simulink library "xps_library"  (R2018a)
settings: Solver=ode45  StartTime=0.0  StopTime=10.0  RelTol=1e-3
undefined symbols (not defined in the file or in its folder): ip_name, lib_path
libraries: xbsIndex_r4 x2454, casper_library_flow_control x68, simulink x52, $bdroot x22, casper_library_misc x9
(part 15 of 27)

== system xps_library/Memory/hmc/sim_mem1 ==
  rd_en : Inport
  wr_en : Inport  Port=2
  wr_addr : Inport  Port=3
  data : Inport  Port=4
  rd_addr : Inport  Port=5
  rd_tag : Inport  Port=6
  Data Type Conversion : DataTypeConversion  OutDataTypeStr=single
  Data Type Conversion2 : DataTypeConversion  OutDataTypeStr=boolean
  Data Type Conversion3 : DataTypeConversion  OutDataTypeStr=single
  Data Type Conversion4 : DataTypeConversion  OutDataTypeStr=boolean
  Data Type Conversion5 : DataTypeConversion  OutDataTypeStr=single
  bus_create : Subsystem  AncestorBlock=casper_library_flow_control/bus_create  mask(bus_create){inputNum=8}
      mask prompts: inputNum "Number of inputs:"
      mask init:
      | bus_create_init(gcb,...
      |     'inputNum', inputNum);
  bus_expand : Subsystem  AncestorBlock=casper_library_flow_control/bus_expand  mask(bus_expand){mode=divisions of equal size, outputNum=8, outputWidth=32, outputBinaryPt=0, outputArithmeticType=0, show_format=off, outputToWorkspace=off, variablePrefix=out, outputToModelAsWell=on}
      mask prompts: outputNum "Number of outputs:"; outputWidth "Output width:"; outputBinaryPt "Output binary point position:"; outputArithmeticType "Output arithmetic type (ufix=0, fix=1, bool=2):"; show_format "Print format string?"; outputToWorkspace "Output to workspace?"; variablePrefix "Variable name prefix:"; outputToModelAsWell "Output to model as well?"
      mask help:
      | Expands a 'bus' made using a bus_create or Xilinx
      | concat block.
      | The input will be divided into the specified number
      | of outputs with the specified arithmetic types.
      | Divisions are made from most significant bit.
      mask init: same as xps_library/IO/forty_gbe/rx_dv_or_exp
      settings: AttributesFormatString=8 outputs
      mask TypeOptions mode: divisions of equal size | divisions of arbitrary size
      mask Callback mode: bus_expand_callback();
      mask Callback outputWidth: bus_expand_callback();
      mask Callback outputToWorkspace: bus_expand_callback();
  data_to_xilinx{1..8} (8 alike) : xbsIndex_r4/Gateway In  gui_display_data_type=Fixed-point  arith_type=Unsigned  n_bits=32  bin_pt=0  preci_type=Single  exp_width=8  frac_width=24  rows=1  columns=1  quantization="Round  (unbiased: +/- Inf)"  overflow=Saturate  period=1  UseAsADC=off  ADCChannel='1'  interface=None  automatic_assignment=on  address_offset=hex2dec('00')  intf_name=''  intf_description=''  default_value=0  timing_constraint=None  locs_specified=off  LOCs={}  io_standard={}  inherit_from_input=off  hdl_port=on  dbl_ovrd=off  block_type=gatewayin
  gateway_data_out : xbsIndex_r4/Gateway Out  inherit_from_input=off  hdl_port=off  rows=1  columns=1  UseAsDAC=off  DACChannel='1'  interface=None  automatic_assignment=on  address_offset=hex2dec('00')  intf_name=''  intf_description=''  timing_constraint=None  locs_specified=off  LOCs={}  io_standard={}  block_type=gatewayout
  sfunc : M-S-Function  FunctionName=hmc_sim_sfunc  Parameters=depth_bits, latency, randread  mask{depth_bits=addr_width, latency=csp_latency, randread=on}
      mask prompts: depth_bits "Depth (2^?):"; latency "Latency (>=1):"; randread "Randomise read results"
      mask init:
      | % if randread
      | %     sprintf('sfunc randread 1')
      | % else
      | %     sprintf('sfunc randread 0')
      | % end
      mask Callback latency:
      | latency = str2double(get_param(gcb, 'latency'));
      | if latency < 1
      |     errordlg('Cannot have latency less than one.');
      |     set_param(gcb, 'latency', '1');
      | end
  sim_data_0_31 : xbsIndex_r4/Gateway Out  inherit_from_input=off  hdl_port=off  rows=1  columns=1  UseAsDAC=off  DACChannel='1'  interface=None  automatic_assignment=on  address_offset=hex2dec('00')  intf_name=''  intf_description=''  timing_constraint=None  locs_specified=off  LOCs={}  io_standard={}  block_type=gatewayout
  sim_data_128_159 : xbsIndex_r4/Gateway Out  inherit_from_input=off  hdl_port=off  rows=1  columns=1  UseAsDAC=off  DACChannel='1'  interface=None  automatic_assignment=on  address_offset=hex2dec('00')  intf_name=''  intf_description=''  timing_constraint=None  locs_specified=off  LOCs={}  io_standard={}  block_type=gatewayout
  sim_data_160_191 : xbsIndex_r4/Gateway Out  inherit_from_input=off  hdl_port=off  rows=1  columns=1  UseAsDAC=off  DACChannel='1'  interface=None  automatic_assignment=on  address_offset=hex2dec('00')  intf_name=''  intf_description=''  timing_constraint=None  locs_specified=off  LOCs={}  io_standard={}  block_type=gatewayout
  sim_data_192_223 : xbsIndex_r4/Gateway Out  inherit_from_input=off  hdl_port=off  rows=1  columns=1  UseAsDAC=off  DACChannel='1'  interface=None  automatic_assignment=on  address_offset=hex2dec('00')  intf_name=''  intf_description=''  timing_constraint=None  locs_specified=off  LOCs={}  io_standard={}  block_type=gatewayout
  sim_data_224_255 : xbsIndex_r4/Gateway Out  inherit_from_input=off  hdl_port=off  rows=1  columns=1  UseAsDAC=off  DACChannel='1'  interface=None  automatic_assignment=on  address_offset=hex2dec('00')  intf_name=''  intf_description=''  timing_constraint=None  locs_specified=off  LOCs={}  io_standard={}  block_type=gatewayout
  sim_data_32_63 : xbsIndex_r4/Gateway Out  inherit_from_input=off  hdl_port=off  rows=1  columns=1  UseAsDAC=off  DACChannel='1'  interface=None  automatic_assignment=on  address_offset=hex2dec('00')  intf_name=''  intf_description=''  timing_constraint=None  locs_specified=off  LOCs={}  io_standard={}  block_type=gatewayout
  sim_data_64_95 : xbsIndex_r4/Gateway Out  inherit_from_input=off  hdl_port=off  rows=1  columns=1  UseAsDAC=off  DACChannel='1'  interface=None  automatic_assignment=on  address_offset=hex2dec('00')  intf_name=''  intf_description=''  timing_constraint=None  locs_specified=off  LOCs={}  io_standard={}  block_type=gatewayout
  sim_data_96_127 : xbsIndex_r4/Gateway Out  inherit_from_input=off  hdl_port=off  rows=1  columns=1  UseAsDAC=off  DACChannel='1'  interface=None  automatic_assignment=on  address_offset=hex2dec('00')  intf_name=''  intf_description=''  timing_constraint=None  locs_specified=off  LOCs={}  io_standard={}  block_type=gatewayout
  sim_rd_addr : xbsIndex_r4/Gateway Out  inherit_from_input=off  hdl_port=off  rows=1  columns=1  UseAsDAC=off  DACChannel='1'  interface=None  automatic_assignment=on  address_offset=hex2dec('00')  intf_name=''  intf_description=''  timing_constraint=None  locs_specified=off  LOCs={}  io_standard={}  block_type=gatewayout
  sim_rd_en : xbsIndex_r4/Gateway Out  inherit_from_input=off  hdl_port=off  rows=1  columns=1  UseAsDAC=off  DACChannel='1'  interface=None  automatic_assignment=on  address_offset=hex2dec('00')  intf_name=''  intf_description=''  timing_constraint=None  locs_specified=off  LOCs={}  io_standard={}  block_type=gatewayout
  sim_rd_tag : xbsIndex_r4/Gateway Out  inherit_from_input=off  hdl_port=off  rows=1  columns=1  UseAsDAC=off  DACChannel='1'  interface=None  automatic_assignment=on  address_offset=hex2dec('00')  intf_name=''  intf_description=''  timing_constraint=None  locs_specified=off  LOCs={}  io_standard={}  block_type=gatewayout
  sim_rw_addr : xbsIndex_r4/Gateway Out  inherit_from_input=off  hdl_port=off  rows=1  columns=1  UseAsDAC=off  DACChannel='1'  interface=None  automatic_assignment=on  address_offset=hex2dec('00')  intf_name=''  intf_description=''  timing_constraint=None  locs_specified=off  LOCs={}  io_standard={}  block_type=gatewayout
  sim_wr_en : xbsIndex_r4/Gateway Out  inherit_from_input=off  hdl_port=off  rows=1  columns=1  UseAsDAC=off  DACChannel='1'  interface=None  automatic_assignment=on  address_offset=hex2dec('00')  intf_name=''  intf_description=''  timing_constraint=None  locs_specified=off  LOCs={}  io_standard={}  block_type=gatewayout
  data_out : Outport
  dv_out : Outport  Port=2
  tag_out : Outport  Port=3
  wires:
  bus_expand/8(lsb_out1) -> sim_data_224_255/1
  bus_expand/7(out2) -> sim_data_192_223/1
  bus_expand/6(out3) -> sim_data_160_191/1
  bus_expand/5(out4) -> sim_data_128_159/1
  bus_expand/4(out5) -> sim_data_96_127/1
  bus_expand/3(out6) -> sim_data_64_95/1
  bus_expand/2(out7) -> sim_data_32_63/1
  bus_expand/1(msb_out8) -> sim_data_0_31/1
  rd_tag/1 -> sim_rd_tag/1
  sim_rd_tag/1 -> Data Type Conversion3/1
  rd_addr/1 -> sim_rd_addr/1
  sim_rd_addr/1 -> Data Type Conversion5/1
  rd_en/1 -> sim_rd_en/1
  sim_rd_en/1 -> Data Type Conversion4/1
  Data Type Conversion4/1 -> sfunc/1  "rd_en"
  wr_addr/1 -> sim_rw_addr/1
  wr_en/1 -> sim_wr_en/1
  sim_rw_addr/1 -> Data Type Conversion/1
  sim_wr_en/1 -> Data Type Conversion2/1
  Data Type Conversion/1 -> sfunc/3  "wr_addr"
  Data Type Conversion2/1 -> sfunc/2  "wr_en"
  Data Type Conversion5/1 -> sfunc/12  "rd_addr"
  Data Type Conversion3/1 -> sfunc/13  "rd_tag"
  data/1 -> bus_expand/1(bus_in)
  sim_data_224_255/1 -> sfunc/11
  sim_data_192_223/1 -> sfunc/10
  sim_data_160_191/1 -> sfunc/9
  sim_data_128_159/1 -> sfunc/8
  sim_data_96_127/1 -> sfunc/7
  sim_data_64_95/1 -> sfunc/6
  sim_data_32_63/1 -> sfunc/5
  sim_data_0_31/1 -> sfunc/4
  bus_create/1(bus_out) -> gateway_data_out/1
  gateway_data_out/1 -> data_out/1
  data_to_xilinx1/1 -> bus_create/1(in1)
  data_to_xilinx2/1 -> bus_create/2(in2)
  data_to_xilinx3/1 -> bus_create/3(in3)
  data_to_xilinx5/1 -> bus_create/5(in5)
  data_to_xilinx6/1 -> bus_create/6(in6)
  data_to_xilinx7/1 -> bus_create/7(in7)
  data_to_xilinx8/1 -> bus_create/8(in8)
  data_to_xilinx4/1 -> bus_create/4(in4)
  sfunc/1 -> data_to_xilinx1/1  "output"
  sfunc/2 -> data_to_xilinx2/1
  sfunc/3 -> data_to_xilinx3/1
  sfunc/4 -> data_to_xilinx4/1
  sfunc/5 -> data_to_xilinx5/1
  sfunc/6 -> data_to_xilinx6/1
  sfunc/7 -> data_to_xilinx7/1
  sfunc/8 -> data_to_xilinx8/1
  sfunc/9 -> dv_out/1
  sfunc/10 -> tag_out/1

== system xps_library/Memory/hmc/sim_mem2 ==
  rd_en : Inport
  wr_en : Inport  Port=2
  wr_addr : Inport  Port=3
  data : Inport  Port=4
  rd_addr : Inport  Port=5
  rd_tag : Inport  Port=6
  Data Type Conversion : DataTypeConversion  OutDataTypeStr=single
  Data Type Conversion2 : DataTypeConversion  OutDataTypeStr=boolean
  Data Type Conversion3 : DataTypeConversion  OutDataTypeStr=single
  Data Type Conversion4 : DataTypeConversion  OutDataTypeStr=boolean
  Data Type Conversion5 : DataTypeConversion  OutDataTypeStr=single
  bus_create : Subsystem  AncestorBlock=casper_library_flow_control/bus_create  mask(bus_create){inputNum=8}
      mask prompts: inputNum "Number of inputs:"
      mask init:
      | bus_create_init(gcb,...
      |     'inputNum', inputNum);
  bus_expand : Subsystem  AncestorBlock=casper_library_flow_control/bus_expand  mask(bus_expand){mode=divisions of equal size, outputNum=8, outputWidth=32, outputBinaryPt=0, outputArithmeticType=0, show_format=off, outputToWorkspace=off, variablePrefix=out, outputToModelAsWell=on}
      mask prompts: outputNum "Number of outputs:"; outputWidth "Output width:"; outputBinaryPt "Output binary point position:"; outputArithmeticType "Output arithmetic type (ufix=0, fix=1, bool=2):"; show_format "Print format string?"; outputToWorkspace "Output to workspace?"; variablePrefix "Variable name prefix:"; outputToModelAsWell "Output to model as well?"
      mask help:
      | Expands a 'bus' made using a bus_create or Xilinx
      | concat block.
      | The input will be divided into the specified number
      | of outputs with the specified arithmetic types.
      | Divisions are made from most significant bit.
      mask init: same as xps_library/IO/forty_gbe/rx_dv_or_exp
      settings: AttributesFormatString=8 outputs
      mask TypeOptions mode: divisions of equal size | divisions of arbitrary size
      mask Callback mode: bus_expand_callback();
      mask Callback outputWidth: bus_expand_callback();
      mask Callback outputToWorkspace: bus_expand_callback();
  data_to_xilinx{1..8} (8 alike) : xbsIndex_r4/Gateway In  gui_display_data_type=Fixed-point  arith_type=Unsigned  n_bits=32  bin_pt=0  preci_type=Single  exp_width=8  frac_width=24  rows=1  columns=1  quantization="Round  (unbiased: +/- Inf)"  overflow=Saturate  period=1  UseAsADC=off  ADCChannel='1'  interface=None  automatic_assignment=on  address_offset=hex2dec('00')  intf_name=''  intf_description=''  default_value=0  timing_constraint=None  locs_specified=off  LOCs={}  io_standard={}  inherit_from_input=off  hdl_port=on  dbl_ovrd=off  block_type=gatewayin
  gateway_data_out : xbsIndex_r4/Gateway Out  inherit_from_input=off  hdl_port=off  rows=1  columns=1  UseAsDAC=off  DACChannel='1'  interface=None  automatic_assignment=on  address_offset=hex2dec('00')  intf_name=''  intf_description=''  timing_constraint=None  locs_specified=off  LOCs={}  io_standard={}  block_type=gatewayout
  sfunc : M-S-Function  FunctionName=hmc_sim_sfunc  Parameters=depth_bits, latency, randread  mask{depth_bits=addr_width, latency=csp_latency, randread=on}
      mask prompts: depth_bits "Depth (2^?):"; latency "Latency (>=1):"; randread "Randomise read results"
      mask Callback latency:
      | latency = str2double(get_param(gcb, 'latency'));
      | if latency < 1
      |     errordlg('Cannot have latency less than one.');
      |     set_param(gcb, 'latency', '1');
      | end
  sim_data_0_31 : xbsIndex_r4/Gateway Out  inherit_from_input=off  hdl_port=off  rows=1  columns=1  UseAsDAC=off  DACChannel='1'  interface=None  automatic_assignment=on  address_offset=hex2dec('00')  intf_name=''  intf_description=''  timing_constraint=None  locs_specified=off  LOCs={}  io_standard={}  block_type=gatewayout
  sim_data_128_159 : xbsIndex_r4/Gateway Out  inherit_from_input=off  hdl_port=off  rows=1  columns=1  UseAsDAC=off  DACChannel='1'  interface=None  automatic_assignment=on  address_offset=hex2dec('00')  intf_name=''  intf_description=''  timing_constraint=None  locs_specified=off  LOCs={}  io_standard={}  block_type=gatewayout
  sim_data_160_191 : xbsIndex_r4/Gateway Out  inherit_from_input=off  hdl_port=off  rows=1  columns=1  UseAsDAC=off  DACChannel='1'  interface=None  automatic_assignment=on  address_offset=hex2dec('00')  intf_name=''  intf_description=''  timing_constraint=None  locs_specified=off  LOCs={}  io_standard={}  block_type=gatewayout
  sim_data_192_223 : xbsIndex_r4/Gateway Out  inherit_from_input=off  hdl_port=off  rows=1  columns=1  UseAsDAC=off  DACChannel='1'  interface=None  automatic_assignment=on  address_offset=hex2dec('00')  intf_name=''  intf_description=''  timing_constraint=None  locs_specified=off  LOCs={}  io_standard={}  block_type=gatewayout
  sim_data_224_255 : xbsIndex_r4/Gateway Out  inherit_from_input=off  hdl_port=off  rows=1  columns=1  UseAsDAC=off  DACChannel='1'  interface=None  automatic_assignment=on  address_offset=hex2dec('00')  intf_name=''  intf_description=''  timing_constraint=None  locs_specified=off  LOCs={}  io_standard={}  block_type=gatewayout
  sim_data_32_63 : xbsIndex_r4/Gateway Out  inherit_from_input=off  hdl_port=off  rows=1  columns=1  UseAsDAC=off  DACChannel='1'  interface=None  automatic_assignment=on  address_offset=hex2dec('00')  intf_name=''  intf_description=''  timing_constraint=None  locs_specified=off  LOCs={}  io_standard={}  block_type=gatewayout
  sim_data_64_95 : xbsIndex_r4/Gateway Out  inherit_from_input=off  hdl_port=off  rows=1  columns=1  UseAsDAC=off  DACChannel='1'  interface=None  automatic_assignment=on  address_offset=hex2dec('00')  intf_name=''  intf_description=''  timing_constraint=None  locs_specified=off  LOCs={}  io_standard={}  block_type=gatewayout
  sim_data_96_127 : xbsIndex_r4/Gateway Out  inherit_from_input=off  hdl_port=off  rows=1  columns=1  UseAsDAC=off  DACChannel='1'  interface=None  automatic_assignment=on  address_offset=hex2dec('00')  intf_name=''  intf_description=''  timing_constraint=None  locs_specified=off  LOCs={}  io_standard={}  block_type=gatewayout
  sim_rd_addr : xbsIndex_r4/Gateway Out  inherit_from_input=off  hdl_port=off  rows=1  columns=1  UseAsDAC=off  DACChannel='1'  interface=None  automatic_assignment=on  address_offset=hex2dec('00')  intf_name=''  intf_description=''  timing_constraint=None  locs_specified=off  LOCs={}  io_standard={}  block_type=gatewayout
  sim_rd_en : xbsIndex_r4/Gateway Out  inherit_from_input=off  hdl_port=off  rows=1  columns=1  UseAsDAC=off  DACChannel='1'  interface=None  automatic_assignment=on  address_offset=hex2dec('00')  intf_name=''  intf_description=''  timing_constraint=None  locs_specified=off  LOCs={}  io_standard={}  block_type=gatewayout
  sim_rd_tag : xbsIndex_r4/Gateway Out  inherit_from_input=off  hdl_port=off  rows=1  columns=1  UseAsDAC=off  DACChannel='1'  interface=None  automatic_assignment=on  address_offset=hex2dec('00')  intf_name=''  intf_description=''  timing_constraint=None  locs_specified=off  LOCs={}  io_standard={}  block_type=gatewayout
  sim_rw_addr : xbsIndex_r4/Gateway Out  inherit_from_input=off  hdl_port=off  rows=1  columns=1  UseAsDAC=off  DACChannel='1'  interface=None  automatic_assignment=on  address_offset=hex2dec('00')  intf_name=''  intf_description=''  timing_constraint=None  locs_specified=off  LOCs={}  io_standard={}  block_type=gatewayout
  sim_wr_en : xbsIndex_r4/Gateway Out  inherit_from_input=off  hdl_port=off  rows=1  columns=1  UseAsDAC=off  DACChannel='1'  interface=None  automatic_assignment=on  address_offset=hex2dec('00')  intf_name=''  intf_description=''  timing_constraint=None  locs_specified=off  LOCs={}  io_standard={}  block_type=gatewayout
  data_out : Outport
  dv_out : Outport  Port=2
  tag_out : Outport  Port=3
  wires:
  bus_expand/8(lsb_out1) -> sim_data_224_255/1
  bus_expand/7(out2) -> sim_data_192_223/1
  bus_expand/6(out3) -> sim_data_160_191/1
  bus_expand/5(out4) -> sim_data_128_159/1
  bus_expand/4(out5) -> sim_data_96_127/1
  bus_expand/3(out6) -> sim_data_64_95/1
  bus_expand/2(out7) -> sim_data_32_63/1
  bus_expand/1(msb_out8) -> sim_data_0_31/1
  rd_tag/1 -> sim_rd_tag/1
  sim_rd_tag/1 -> Data Type Conversion3/1
  rd_addr/1 -> sim_rd_addr/1
  sim_rd_addr/1 -> Data Type Conversion5/1
  rd_en/1 -> sim_rd_en/1
  sim_rd_en/1 -> Data Type Conversion4/1
  Data Type Conversion4/1 -> sfunc/1  "rd_en"
  wr_addr/1 -> sim_rw_addr/1
  wr_en/1 -> sim_wr_en/1
  sim_rw_addr/1 -> Data Type Conversion/1
  sim_wr_en/1 -> Data Type Conversion2/1
  Data Type Conversion/1 -> sfunc/3  "wr_addr"
  Data Type Conversion2/1 -> sfunc/2  "wr_en"
  Data Type Conversion5/1 -> sfunc/12  "rd_addr"
  Data Type Conversion3/1 -> sfunc/13  "rd_tag"
  data/1 -> bus_expand/1(bus_in)
  sim_data_224_255/1 -> sfunc/11
  sim_data_192_223/1 -> sfunc/10
  sim_data_160_191/1 -> sfunc/9
  sim_data_128_159/1 -> sfunc/8
  sim_data_96_127/1 -> sfunc/7
  sim_data_64_95/1 -> sfunc/6
  sim_data_32_63/1 -> sfunc/5
  sim_data_0_31/1 -> sfunc/4
  gateway_data_out/1 -> data_out/1
  bus_create/1(bus_out) -> gateway_data_out/1
  data_to_xilinx1/1 -> bus_create/1(in1)
  data_to_xilinx2/1 -> bus_create/2(in2)
  data_to_xilinx3/1 -> bus_create/3(in3)
  data_to_xilinx5/1 -> bus_create/5(in5)
  data_to_xilinx6/1 -> bus_create/6(in6)
  data_to_xilinx7/1 -> bus_create/7(in7)
  data_to_xilinx8/1 -> bus_create/8(in8)
  data_to_xilinx4/1 -> bus_create/4(in4)
  sfunc/1 -> data_to_xilinx1/1  "output"
  sfunc/2 -> data_to_xilinx2/1
  sfunc/3 -> data_to_xilinx3/1
  sfunc/4 -> data_to_xilinx4/1
  sfunc/5 -> data_to_xilinx5/1
  sfunc/6 -> data_to_xilinx6/1
  sfunc/7 -> data_to_xilinx7/1
  sfunc/8 -> data_to_xilinx8/1
  sfunc/9 -> dv_out/1
  sfunc/10 -> tag_out/1

== system xps_library/Memory/qdr/qdr_sim_model ==
  rd_en : Inport
  wr_en : Inport  Port=2
  be : Inport  Port=3
  addr : Inport  Port=4
  data_in : Inport  Port=5
  AddSub : xbsIndex_r4/AddSub  mode=Addition  use_carryin=off  use_carryout=off  en=off  latency=0  precision=Full  arith_type=Unsigned  n_bits=16  bin_pt=14  quantization=Truncate  overflow=Wrap  use_behavioral_HDL=off  hw_selection=Fabric  pipelined=off  use_rpm=on  dbl_ovrd=off  block_type=addsub
      settings: block_version=10.1.3
  Concat : xbsIndex_r4/Concat  num_inputs=2  dbl_ovrd=off  block_type=concat
      settings: block_version=10.1.3
  Constant1 : xbsIndex_r4/Constant  const=0  gui_display_data_type=Fixed-point  arith_type=Unsigned  n_bits=1  bin_pt=0  preci_type=Single  exp_width=8  frac_width=24  explicit_period=on  period=1  equ=P=C  opselect=C  inp2=PCIN>>17  opr=+  inp1=P  carry=CIN  dbl_ovrd=off  block_type=constant
  Constant2 : xbsIndex_r4/Constant  const=1  gui_display_data_type=Fixed-point  arith_type=Unsigned  n_bits=33  bin_pt=0  preci_type=Single  exp_width=8  frac_width=24  explicit_period=on  period=1  equ=P=C  opselect=C  inp2=PCIN>>17  opr=+  inp1=P  carry=CIN  dbl_ovrd=off  block_type=constant
  Delay : xbsIndex_r4/Delay  rst=off  infoeditControl=Selection of Reset will increase slice count due to use of real FFs and instead of SRLs  en=off  latency=9  reg_retiming=off  dbl_ovrd=off  block_type=delay
  Delay{1..3,5} (4 alike) : xbsIndex_r4/Delay  rst=off  infoeditControl=Selection of Reset will increase slice count due to use of real FFs and instead of SRLs  en=off  latency=1  reg_retiming=off  dbl_ovrd=off  block_type=delay
  Delay4 : xbsIndex_r4/Delay  rst=off  infoeditControl=Selection of Reset will increase slice count due to use of real FFs and instead of SRLs  en=off  latency=10  reg_retiming=off  dbl_ovrd=off  block_type=delay
  Dual Port RAM : xbsIndex_r4/Dual Port RAM  depth=2^qdr_awidth  initVector=[1:2^qdr_awidth]  distributed_mem=Block RAM  init_a=0  init_b=0  rst_a=off  rst_b=off  en_a=off  en_b=off  latency=1  write_mode_A=Read After Write  write_mode_B=Read After Write  optimize=Area  dbl_ovrd=off  block_type=dpram
      settings: block_version=10.1.3
  Inverter1 : xbsIndex_r4/Inverter  en=off  latency=0  dbl_ovrd=off  block_type=inv
  Inverter2 : xbsIndex_r4/Inverter  en=off  latency=0  dbl_ovrd=off  block_type=inv
  Inverter3 : xbsIndex_r4/Inverter  en=off  latency=0  dbl_ovrd=off  block_type=inv
  Logical : xbsIndex_r4/Logical  logical_function=AND  inputs=2  en=off  latency=0  precision=Full  arith_type=Unsigned  n_bits=16  bin_pt=0  align_bp=on  dbl_ovrd=off  block_type=logical
  Logical1 : xbsIndex_r4/Logical  logical_function=AND  inputs=2  en=off  latency=0  precision=Full  arith_type=Unsigned  n_bits=16  bin_pt=0  align_bp=on  dbl_ovrd=off  block_type=logical
  Logical2 : xbsIndex_r4/Logical  logical_function=AND  inputs=2  en=off  latency=0  precision=Full  arith_type=Unsigned  n_bits=16  bin_pt=0  align_bp=on  dbl_ovrd=off  block_type=logical
  Logical3 : xbsIndex_r4/Logical  logical_function=OR  inputs=2  en=off  latency=0  precision=Full  arith_type=Unsigned  n_bits=16  bin_pt=0  align_bp=on  dbl_ovrd=off  block_type=logical
  Mux : xbsIndex_r4/Mux  inputs=2  en=off  latency=0  precision=Full  arith_type=Unsigned  n_bits=16  bin_pt=14  quantization=Truncate  overflow=Wrap  dbl_ovrd=off  block_type=mux
  Terminator : Terminator
  convert_address : xbsIndex_r4/Convert  gui_display_data_type=Fixed-point  arith_type=Unsigned  n_bits=qdr_awidth  bin_pt=0  float_type=Single  exp_bits=8  fraction_bits=24  quantization=Truncate  overflow=Wrap  en=off  latency=0  pipeline=off  dbl_ovrd=off  block_type=convert
      settings: xl_area=[0, 0, 0, 0, 0, 0, 0]
  convert_address1 : xbsIndex_r4/Convert  gui_display_data_type=Fixed-point  arith_type=Unsigned  n_bits=qdr_awidth  bin_pt=0  float_type=Single  exp_bits=8  fraction_bits=24  quantization=Truncate  overflow=Wrap  en=off  latency=0  pipeline=off  dbl_ovrd=off  block_type=convert
      settings: xl_area=[0, 0, 0, 0, 0, 0, 0]
  prev_rd : xbsIndex_r4/Register  init=0  rst=off  en=off  dbl_ovrd=off  block_type=register
  prev_w : xbsIndex_r4/Register  init=0  rst=off  en=off  dbl_ovrd=off  block_type=register
  sim_data_out : xbsIndex_r4/Gateway Out  inherit_from_input=off  hdl_port=off  rows=1  columns=1  UseAsDAC=off  DACChannel='1'  interface=None  automatic_assignment=on  address_offset=hex2dec('00')  intf_name=''  intf_description=''  timing_constraint=None  locs_specified=off  LOCs={'B21','B22','A22','B23','B19','C19','A20','A21','A23','B24','A24','A25','E18','D18','C18','B18'}  io_standard={}  block_type=gatewayout
      settings: sginterface={'Nallatech'=>{'xdspkit'=>{'non_memory_mapped_port'=>'sim_data_out'}},'Xilinx'=>{'jtaghwcosim'=>{'non_memory_mapped_port'=>'sim_data_out'},'xdspkit'=>{'non_memory_mapped_port'=>'sim_data_out'}}}  xl_area=[0, 0, 0, 0, 0, 0, 0]
  sim_data_vld : xbsIndex_r4/Gateway Out  inherit_from_input=off  hdl_port=off  rows=1  columns=1  UseAsDAC=off  DACChannel='1'  interface=None  automatic_assignment=on  address_offset=hex2dec('00')  intf_name=''  intf_description=''  timing_constraint=None  locs_specified=off  LOCs={'B21','B22','A22','B23','B19','C19','A20','A21','A23','B24','A24','A25','E18','D18','C18','B18'}  io_standard={}  block_type=gatewayout
      settings: sginterface={'Nallatech'=>{'xdspkit'=>{'non_memory_mapped_port'=>'sim_data_out'}},'Xilinx'=>{'jtaghwcosim'=>{'non_memory_mapped_port'=>'sim_data_out'},'xdspkit'=>{'non_memory_mapped_port'=>'sim_data_out'}}}  xl_area=[0, 0, 0, 0, 0, 0, 0]
  data_out : Outport
  data_valid : Outport  Port=2
  wires:
  Dual Port RAM/2 -> Mux/2
  Dual Port RAM/1 -> Mux/3
  Delay3/1 -> Mux/1
  [R] -> Delay3/1
  Mux/1 -> Delay/1
  Inverter1/1 -> Logical1/2
  Inverter3/1 -> Logical2/2
  Logical2/1 -> prev_w/1, [W]
  prev_w/1 -> Inverter3/1
  Logical1/1 -> Logical2/1
  [W] -> Delay1/1
  [W] -> Dual Port RAM/3
  [A] -> convert_address/1
  [Az] -> convert_address1/1
  [D] -> Dual Port RAM/2
  data_in/1 -> [D]
  [R] -> Inverter1/1
  wr_en/1 -> Logical1/1
  Logical/1 -> [R], prev_rd/1
  Inverter2/1 -> Logical/2
  prev_rd/1 -> Inverter2/1
  rd_en/1 -> Delay4/1, Logical/1
  AddSub/1 -> [Az]
  Constant2/1 -> AddSub/2
  Delay2/1 -> AddSub/1
  Concat/1 -> [A], Delay2/1
  Constant1/1 -> Concat/2
  addr/1 -> Concat/1
  Delay1/1 -> Dual Port RAM/6
  [D] -> Dual Port RAM/5
  convert_address/1 -> Dual Port RAM/1
  convert_address1/1 -> Dual Port RAM/4
  sim_data_out/1 -> data_out/1
  Delay/1 -> sim_data_out/1
  be/1 -> Terminator/1
  sim_data_vld/1 -> data_valid/1
  Delay4/1 -> Delay5/1, Logical3/1
  Delay5/1 -> Logical3/2
  Logical3/1 -> sim_data_vld/1

== system xps_library/Memory/shared_bram/calc_add ==
  note: If reading/writing words
      | smaller than 32 bits,
      | change address so
      | that addressing is
      | big endian instead of
      | little, otherwise
      | pass through
  note: Use behavioural HDL
      | so that gets optimised
      | to minimum logic
  in : Inport
  add_sub : xbsIndex_r4/AddSub  mode=Subtraction  use_carryin=off  use_carryout=off  en=off  latency=0  precision=User Defined  arith_type=Unsigned  n_bits=max(1, log2(32/data_width))  bin_pt=0  quantization=Truncate  overflow=Wrap  use_behavioral_HDL=on  hw_selection=Fabric  pipelined=off  dbl_ovrd=off  block_type=addsub
  concat : xbsIndex_r4/Concat  num_inputs=2  dbl_ovrd=off  block_type=concat
  const : xbsIndex_r4/Constant  const=max(0, 32/data_width-1)  gui_display_data_type=Fixed-point  arith_type=Unsigned  n_bits=max(1, log2(32/data_width))  bin_pt=0  preci_type=Single  exp_width=8  frac_width=24  explicit_period=on  period=sample_rate  equ=P=C  opselect=C  inp2=PCIN>>17  opr=+  inp1=P  carry=CIN  dbl_ovrd=off  block_type=constant
      settings: block_version=11.4
  convert_addr : xbsIndex_r4/Convert  gui_display_data_type=Fixed-point  arith_type=Unsigned  n_bits=addr_width  bin_pt=0  float_type=Single  exp_bits=8  fraction_bits=24  quantization=Truncate  overflow=Wrap  en=off  latency=0  pipeline=off  dbl_ovrd=off  block_type=convert
      settings: xl_area=[0, 0, 0, 0, 0, 0, 0]
  lsw : xbsIndex_r4/Slice  nbits=max(1, log2(32/data_width))  boolean_output=off  mode=Lower Bit Location + Width  bit1=0  base1=MSB of Input  bit0=0  base0=LSB of Input  dbl_ovrd=off  block_type=slice
  manipulate : xbsIndex_r4/Constant  const=min(1, floor(32/data_width) - 1)  gui_display_data_type=Fixed-point  arith_type=Unsigned  n_bits=1  bin_pt=0  preci_type=Single  exp_width=8  frac_width=24  explicit_period=on  period=sample_rate  equ=P=C  opselect=C  inp2=PCIN>>17  opr=+  inp1=P  carry=CIN  dbl_ovrd=off  block_type=constant
      settings: block_version=11.4
  msw : xbsIndex_r4/Slice  nbits=addr_width - max(1, log2(32/data_width))  boolean_output=off  mode=Upper Bit Location + Width  bit1=0  base1=MSB of Input  bit0=0  base0=LSB of Input  dbl_ovrd=off  block_type=slice
  mux : xbsIndex_r4/Mux  inputs=2  en=off  latency=0  precision=Full  arith_type=Unsigned  n_bits=16  bin_pt=14  quantization=Truncate  overflow=Wrap  dbl_ovrd=off  block_type=mux
      settings: block_version=11.4
  out : Outport
  wires:
  in/1 -> convert_addr/1
  add_sub/1 -> concat/2
  msw/1 -> concat/1
  concat/1 -> mux/3
  manipulate/1 -> mux/1
  mux/1 -> out/1
  lsw/1 -> add_sub/2
  const/1 -> add_sub/1
  convert_addr/1 -> lsw/1, msw/1, mux/2

== system xps_library/Memory/shared_bram/munge_in ==
  din : Inport
  reinterpret_out : xbsIndex_r4/Reinterpret  force_arith_type=on  arith_type=Unsigned  force_bin_pt=on  bin_pt=0  block_type=reinterpret
  dout : Outport
  wires:
  reinterpret_out/1 -> dout/1
  din/1 -> reinterpret_out/1

== system xps_library/Memory/shared_bram/munge_out ==
  din : Inport
  reinterpret_out : xbsIndex_r4/Reinterpret  force_arith_type=on  arith_type=Unsigned  force_bin_pt=on  bin_pt=0  block_type=reinterpret
  dout : Outport
  wires:
  reinterpret_out/1 -> dout/1
  din/1 -> reinterpret_out/1

== system xps_library/Memory/shared_bram/sim_mem ==
  addr : Inport
  data : Inport  Port=2
  we : Inport  Port=3
  Data Type Conversion : DataTypeConversion  OutDataTypeStr=single
  Data Type Conversion1 : DataTypeConversion  OutDataTypeStr=double
  Data Type Conversion2 : DataTypeConversion  OutDataTypeStr=boolean
  sfunc : M-S-Function  FunctionName=shared_bram_sim_sfunc  Parameters=depth_bits, latency, init_vals  mask{depth_bits=addr_width, latency=csp_latency, init_vals=init_vals}
      mask prompts: depth_bits "Depth (2^?):"; latency "Latency (>=1):"; init_vals "Initial values:"
      mask Callback latency:
      | latency = str2double(get_param(gcb, 'latency'));
      | if latency < 1
      |     errordlg('Cannot have latency less than one.');
      |     set_param(gcb, 'latency', '1');
      | end
  sim_addr : xbsIndex_r4/Gateway Out  inherit_from_input=off  hdl_port=off  rows=1  columns=1  UseAsDAC=off  DACChannel='1'  interface=None  automatic_assignment=on  address_offset=hex2dec('00')  intf_name=''  intf_description=''  timing_constraint=None  locs_specified=off  LOCs={}  io_standard={}  block_type=gatewayout
  sim_data : xbsIndex_r4/Gateway Out  inherit_from_input=off  hdl_port=off  rows=1  columns=1  UseAsDAC=off  DACChannel='1'  interface=None  automatic_assignment=on  address_offset=hex2dec('00')  intf_name=''  intf_description=''  timing_constraint=None  locs_specified=off  LOCs={}  io_standard={}  block_type=gatewayout
  sim_we : xbsIndex_r4/Gateway Out  inherit_from_input=off  hdl_port=off  rows=1  columns=1  UseAsDAC=off  DACChannel='1'  interface=None  automatic_assignment=on  address_offset=hex2dec('00')  intf_name=''  intf_description=''  timing_constraint=None  locs_specified=off  LOCs={}  io_standard={}  block_type=gatewayout
  data_out : Outport
  wires:
  addr/1 -> sim_addr/1
  data/1 -> sim_data/1
  we/1 -> sim_we/1
  sim_addr/1 -> Data Type Conversion/1
  sim_data/1 -> Data Type Conversion1/1
  sim_we/1 -> Data Type Conversion2/1
  Data Type Conversion/1 -> sfunc/1  "addr"
  Data Type Conversion1/1 -> sfunc/2  "data_in"
  Data Type Conversion2/1 -> sfunc/3  "we"
  sfunc/1 -> data_out/1  "output"

== system xps_library/DACs/dac_mkid/Subsystem/parallel_to_serial_converter ==
  pin : Inport
  ld : Inport  Port=2
  shift : Inport  Port=3
  Logical : xbsIndex_r4/Logical  logical_function=OR  inputs=2  en=off  latency=0  precision=Full  arith_type=Unsigned  n_bits=16  bin_pt=0  align_bp=on  dbl_ovrd=off  block_type=logical
  filler : xbsIndex_r4/Constant  const=0  gui_display_data_type=Fixed-point  arith_type=Unsigned  n_bits=sout_width  bin_pt=0  preci_type=Single  exp_width=8  frac_width=24  explicit_period=on  period=1  equ=P=C  opselect=C  inp2=PCIN>>17  opr=+  inp1=P  carry=CIN  dbl_ovrd=off  block_type=constant
  shifter_unit1 : casper_library_flow_control/shifter_unit  data_width=1  pin_offset=0
      settings: SourceProductName=CASPER DSP Blockset
  shifter_unit10 : casper_library_flow_control/shifter_unit  data_width=1  pin_offset=9
      settings: SourceProductName=CASPER DSP Blockset
  shifter_unit11 : casper_library_flow_control/shifter_unit  data_width=1  pin_offset=10
      settings: SourceProductName=CASPER DSP Blockset
  shifter_unit12 : casper_library_flow_control/shifter_unit  data_width=1  pin_offset=11
      settings: SourceProductName=CASPER DSP Blockset
  shifter_unit13 : casper_library_flow_control/shifter_unit  data_width=1  pin_offset=12
      settings: SourceProductName=CASPER DSP Blockset
  shifter_unit14 : casper_library_flow_control/shifter_unit  data_width=1  pin_offset=13
      settings: SourceProductName=CASPER DSP Blockset
  shifter_unit15 : casper_library_flow_control/shifter_unit  data_width=1  pin_offset=14
      settings: SourceProductName=CASPER DSP Blockset
  shifter_unit16 : casper_library_flow_control/shifter_unit  data_width=1  pin_offset=15
      settings: SourceProductName=CASPER DSP Blockset
  shifter_unit17 : casper_library_flow_control/shifter_unit  data_width=1  pin_offset=16
      settings: SourceProductName=CASPER DSP Blockset
  shifter_unit2 : casper_library_flow_control/shifter_unit  data_width=1  pin_offset=1
      settings: SourceProductName=CASPER DSP Blockset
  shifter_unit3 : casper_library_flow_control/shifter_unit  data_width=1  pin_offset=2
      settings: SourceProductName=CASPER DSP Blockset
  shifter_unit4 : casper_library_flow_control/shifter_unit  data_width=1  pin_offset=3
      settings: SourceProductName=CASPER DSP Blockset
  shifter_unit5 : casper_library_flow_control/shifter_unit  data_width=1  pin_offset=4
      settings: SourceProductName=CASPER DSP Blockset
  shifter_unit6 : casper_library_flow_control/shifter_unit  data_width=1  pin_offset=5
      settings: SourceProductName=CASPER DSP Blockset
  shifter_unit7 : casper_library_flow_control/shifter_unit  data_width=1  pin_offset=6
      settings: SourceProductName=CASPER DSP Blockset
  shifter_unit8 : casper_library_flow_control/shifter_unit  data_width=1  pin_offset=7
      settings: SourceProductName=CASPER DSP Blockset
  shifter_unit9 : casper_library_flow_control/shifter_unit  data_width=1  pin_offset=8
      settings: SourceProductName=CASPER DSP Blockset
  sout : Outport
  wires:
  ld/1 -> Logical/1, shifter_unit1/1, shifter_unit2/1, shifter_unit3/1, shifter_unit4/1, shifter_unit5/1, shifter_unit6/1, shifter_unit7/1, shifter_unit8/1, shifter_unit9/1, shifter_unit10/1, shifter_unit11/1, shifter_unit12/1, shifter_unit13/1, shifter_unit14/1, shifter_unit15/1, shifter_unit16/1, shifter_unit17/1
  shift/1 -> Logical/2
  filler/1 -> shifter_unit1/2
  pin/1 -> shifter_unit1/3, shifter_unit2/3, shifter_unit3/3, shifter_unit4/3, shifter_unit5/3, shifter_unit6/3, shifter_unit7/3, shifter_unit8/3, shifter_unit9/3, shifter_unit10/3, shifter_unit11/3, shifter_unit12/3, shifter_unit13/3, shifter_unit14/3, shifter_unit15/3, shifter_unit16/3, shifter_unit17/3
  Logical/1 -> shifter_unit1/4, shifter_unit2/4, shifter_unit3/4, shifter_unit4/4, shifter_unit5/4, shifter_unit6/4, shifter_unit7/4, shifter_unit8/4, shifter_unit9/4, shifter_unit10/4, shifter_unit11/4, shifter_unit12/4, shifter_unit13/4, shifter_unit14/4, shifter_unit15/4, shifter_unit16/4, shifter_unit17/4
  shifter_unit1/1 -> shifter_unit2/2
  shifter_unit2/1 -> shifter_unit3/2
  shifter_unit3/1 -> shifter_unit4/2
  shifter_unit4/1 -> shifter_unit5/2
  shifter_unit5/1 -> shifter_unit6/2
  shifter_unit6/1 -> shifter_unit7/2
  shifter_unit7/1 -> shifter_unit8/2
  shifter_unit8/1 -> shifter_unit9/2
  shifter_unit9/1 -> shifter_unit10/2
  shifter_unit10/1 -> shifter_unit11/2
  shifter_unit11/1 -> shifter_unit12/2
  shifter_unit12/1 -> shifter_unit13/2
  shifter_unit13/1 -> shifter_unit14/2
  shifter_unit14/1 -> shifter_unit15/2
  shifter_unit15/1 -> shifter_unit16/2
  shifter_unit16/1 -> shifter_unit17/2
  shifter_unit17/1 -> sout/1

== system xps_library/DACs/dac_mkid/Subsystem/parallel_to_serial_converter1 ==
  pin : Inport
  ld : Inport  Port=2
  shift : Inport  Port=3
  Logical : xbsIndex_r4/Logical  logical_function=OR  inputs=2  en=off  latency=0  precision=Full  arith_type=Unsigned  n_bits=16  bin_pt=0  align_bp=on  dbl_ovrd=off  block_type=logical
  filler : xbsIndex_r4/Constant  const=0  gui_display_data_type=Fixed-point  arith_type=Unsigned  n_bits=sout_width  bin_pt=0  preci_type=Single  exp_width=8  frac_width=24  explicit_period=on  period=1  equ=P=C  opselect=C  inp2=PCIN>>17  opr=+  inp1=P  carry=CIN  dbl_ovrd=off  block_type=constant
  shifter_unit1 : casper_library_flow_control/shifter_unit  data_width=1  pin_offset=0
      settings: SourceProductName=CASPER DSP Blockset
  shifter_unit10 : casper_library_flow_control/shifter_unit  data_width=1  pin_offset=9
      settings: SourceProductName=CASPER DSP Blockset
  shifter_unit11 : casper_library_flow_control/shifter_unit  data_width=1  pin_offset=10
      settings: SourceProductName=CASPER DSP Blockset
  shifter_unit12 : casper_library_flow_control/shifter_unit  data_width=1  pin_offset=11
      settings: SourceProductName=CASPER DSP Blockset
  shifter_unit13 : casper_library_flow_control/shifter_unit  data_width=1  pin_offset=12
      settings: SourceProductName=CASPER DSP Blockset
  shifter_unit14 : casper_library_flow_control/shifter_unit  data_width=1  pin_offset=13
      settings: SourceProductName=CASPER DSP Blockset
  shifter_unit15 : casper_library_flow_control/shifter_unit  data_width=1  pin_offset=14
      settings: SourceProductName=CASPER DSP Blockset
  shifter_unit16 : casper_library_flow_control/shifter_unit  data_width=1  pin_offset=15
      settings: SourceProductName=CASPER DSP Blockset
  shifter_unit17 : casper_library_flow_control/shifter_unit  data_width=1  pin_offset=16
      settings: SourceProductName=CASPER DSP Blockset
  shifter_unit2 : casper_library_flow_control/shifter_unit  data_width=1  pin_offset=1
      settings: SourceProductName=CASPER DSP Blockset
  shifter_unit3 : casper_library_flow_control/shifter_unit  data_width=1  pin_offset=2
      settings: SourceProductName=CASPER DSP Blockset
  shifter_unit4 : casper_library_flow_control/shifter_unit  data_width=1  pin_offset=3
      settings: SourceProductName=CASPER DSP Blockset
  shifter_unit5 : casper_library_flow_control/shifter_unit  data_width=1  pin_offset=4
      settings: SourceProductName=CASPER DSP Blockset
  shifter_unit6 : casper_library_flow_control/shifter_unit  data_width=1  pin_offset=5
      settings: SourceProductName=CASPER DSP Blockset
  shifter_unit7 : casper_library_flow_control/shifter_unit  data_width=1  pin_offset=6
      settings: SourceProductName=CASPER DSP Blockset
  shifter_unit8 : casper_library_flow_control/shifter_unit  data_width=1  pin_offset=7
      settings: SourceProductName=CASPER DSP Blockset
  shifter_unit9 : casper_library_flow_control/shifter_unit  data_width=1  pin_offset=8
      settings: SourceProductName=CASPER DSP Blockset
  sout : Outport
  wires:
  ld/1 -> Logical/1, shifter_unit1/1, shifter_unit2/1, shifter_unit3/1, shifter_unit4/1, shifter_unit5/1, shifter_unit6/1, shifter_unit7/1, shifter_unit8/1, shifter_unit9/1, shifter_unit10/1, shifter_unit11/1, shifter_unit12/1, shifter_unit13/1, shifter_unit14/1, shifter_unit15/1, shifter_unit16/1, shifter_unit17/1
  shift/1 -> Logical/2
  filler/1 -> shifter_unit1/2
  pin/1 -> shifter_unit1/3, shifter_unit2/3, shifter_unit3/3, shifter_unit4/3, shifter_unit5/3, shifter_unit6/3, shifter_unit7/3, shifter_unit8/3, shifter_unit9/3, shifter_unit10/3, shifter_unit11/3, shifter_unit12/3, shifter_unit13/3, shifter_unit14/3, shifter_unit15/3, shifter_unit16/3, shifter_unit17/3
  Logical/1 -> shifter_unit1/4, shifter_unit2/4, shifter_unit3/4, shifter_unit4/4, shifter_unit5/4, shifter_unit6/4, shifter_unit7/4, shifter_unit8/4, shifter_unit9/4, shifter_unit10/4, shifter_unit11/4, shifter_unit12/4, shifter_unit13/4, shifter_unit14/4, shifter_unit15/4, shifter_unit16/4, shifter_unit17/4
  shifter_unit1/1 -> shifter_unit2/2
  shifter_unit2/1 -> shifter_unit3/2
  shifter_unit3/1 -> shifter_unit4/2
  shifter_unit4/1 -> shifter_unit5/2
  shifter_unit5/1 -> shifter_unit6/2
  shifter_unit6/1 -> shifter_unit7/2
  shifter_unit7/1 -> shifter_unit8/2
  shifter_unit8/1 -> shifter_unit9/2
  shifter_unit9/1 -> shifter_unit10/2
  shifter_unit10/1 -> shifter_unit11/2
  shifter_unit11/1 -> shifter_unit12/2
  shifter_unit12/1 -> shifter_unit13/2
  shifter_unit13/1 -> shifter_unit14/2
  shifter_unit14/1 -> shifter_unit15/2
  shifter_unit15/1 -> shifter_unit16/2
  shifter_unit16/1 -> shifter_unit17/2
  shifter_unit17/1 -> sout/1

== system xps_library/DACs/dac_mkid/Subsystem/posedge1 ==
  In : Inport
  Delay : xbsIndex_r4/Delay  rst=off  infoeditControl=Selection of Reset will increase slice count due to use of real FFs and instead of SRLs  en=off  latency=1  reg_retiming=off  dbl_ovrd=off  block_type=delay
      settings: xl_area=[0, 0, 0, 0, 0, 0, 0]  block_version=9.1.01
  Inverter : xbsIndex_r4/Inverter  en=off  latency=0  dbl_ovrd=off  block_type=inv
      settings: xl_area=[0, 0, 0, 0, 0, 0, 0]  block_version=9.1.01
  Logical : xbsIndex_r4/Logical  logical_function=AND  inputs=2  en=off  latency=0  precision=Full  arith_type=Unsigned  n_bits=8  bin_pt=2  align_bp=on  dbl_ovrd=off  block_type=logical
      settings: xl_area=[0, 0, 0, 0, 0, 0, 0]  block_version=9.1.01
  Out : Outport
  wires:
  Delay/1 -> Inverter/1
  Inverter/1 -> Logical/1
  In/1 -> Delay/1, Logical/2
  Logical/1 -> Out/1

== system xps_library/DACs/dac_mkid/Subsystem/posedge2 ==
  In : Inport
  Delay : xbsIndex_r4/Delay  rst=off  infoeditControl=Selection of Reset will increase slice count due to use of real FFs and instead of SRLs  en=off  latency=1  reg_retiming=off  dbl_ovrd=off  block_type=delay
      settings: xl_area=[0, 0, 0, 0, 0, 0, 0]  block_version=9.1.01
  Inverter : xbsIndex_r4/Inverter  en=off  latency=0  dbl_ovrd=off  block_type=inv
      settings: xl_area=[0, 0, 0, 0, 0, 0, 0]  block_version=9.1.01
  Logical : xbsIndex_r4/Logical  logical_function=AND  inputs=2  en=off  latency=0  precision=Full  arith_type=Unsigned  n_bits=8  bin_pt=2  align_bp=on  dbl_ovrd=off  block_type=logical
      settings: xl_area=[0, 0, 0, 0, 0, 0, 0]  block_version=9.1.01
  Out : Outport
  wires:
  Delay/1 -> Inverter/1
  Inverter/1 -> Logical/1
  In/1 -> Delay/1, Logical/2
  Logical/1 -> Out/1

== system xps_library/DACs/dac_mkid/Subsystem/posedge3 ==
  In : Inport
  Delay : xbsIndex_r4/Delay  rst=off  infoeditControl=Selection of Reset will increase slice count due to use of real FFs and instead of SRLs  en=off  latency=1  reg_retiming=off  dbl_ovrd=off  block_type=delay
      settings: xl_area=[0, 0, 0, 0, 0, 0, 0]  block_version=9.1.01
  Inverter : xbsIndex_r4/Inverter  en=off  latency=0  dbl_ovrd=off  block_type=inv
      settings: xl_area=[0, 0, 0, 0, 0, 0, 0]  block_version=9.1.01
  Logical : xbsIndex_r4/Logical  logical_function=AND  inputs=2  en=off  latency=0  precision=Full  arith_type=Unsigned  n_bits=8  bin_pt=2  align_bp=on  dbl_ovrd=off  block_type=logical
      settings: xl_area=[0, 0, 0, 0, 0, 0, 0]  block_version=9.1.01
  Out : Outport
  wires:
  Delay/1 -> Inverter/1
  Inverter/1 -> Logical/1
  In/1 -> Delay/1, Logical/2
  Logical/1 -> Out/1

== system xps_library/DACs/dac_mkid_4x/Subsystem/parallel_to_serial_converter ==
  pin : Inport
  ld : Inport  Port=2
  shift : Inport  Port=3
  Logical : xbsIndex_r4/Logical  logical_function=OR  inputs=2  en=off  latency=0  precision=Full  arith_type=Unsigned  n_bits=16  bin_pt=0  align_bp=on  dbl_ovrd=off  block_type=logical
  filler : xbsIndex_r4/Constant  const=0  gui_display_data_type=Fixed-point  arith_type=Unsigned  n_bits=sout_width  bin_pt=0  preci_type=Single  exp_width=8  frac_width=24  explicit_period=on  period=1  equ=P=C  opselect=C  inp2=PCIN>>17  opr=+  inp1=P  carry=CIN  dbl_ovrd=off  block_type=constant
  shifter_unit1 : casper_library_flow_control/shifter_unit  data_width=1  pin_offset=0
      settings: SourceProductName=CASPER DSP Blockset
  shifter_unit10 : casper_library_flow_control/shifter_unit  data_width=1  pin_offset=9
      settings: SourceProductName=CASPER DSP Blockset
  shifter_unit11 : casper_library_flow_control/shifter_unit  data_width=1  pin_offset=10
      settings: SourceProductName=CASPER DSP Blockset
  shifter_unit12 : casper_library_flow_control/shifter_unit  data_width=1  pin_offset=11
      settings: SourceProductName=CASPER DSP Blockset
  shifter_unit13 : casper_library_flow_control/shifter_unit  data_width=1  pin_offset=12
      settings: SourceProductName=CASPER DSP Blockset
  shifter_unit14 : casper_library_flow_control/shifter_unit  data_width=1  pin_offset=13
      settings: SourceProductName=CASPER DSP Blockset
  shifter_unit15 : casper_library_flow_control/shifter_unit  data_width=1  pin_offset=14
      settings: SourceProductName=CASPER DSP Blockset
  shifter_unit16 : casper_library_flow_control/shifter_unit  data_width=1  pin_offset=15
      settings: SourceProductName=CASPER DSP Blockset
  shifter_unit17 : casper_library_flow_control/shifter_unit  data_width=1  pin_offset=16
      settings: SourceProductName=CASPER DSP Blockset
  shifter_unit2 : casper_library_flow_control/shifter_unit  data_width=1  pin_offset=1
      settings: SourceProductName=CASPER DSP Blockset
  shifter_unit3 : casper_library_flow_control/shifter_unit  data_width=1  pin_offset=2
      settings: SourceProductName=CASPER DSP Blockset
  shifter_unit4 : casper_library_flow_control/shifter_unit  data_width=1  pin_offset=3
      settings: SourceProductName=CASPER DSP Blockset
  shifter_unit5 : casper_library_flow_control/shifter_unit  data_width=1  pin_offset=4
      settings: SourceProductName=CASPER DSP Blockset
  shifter_unit6 : casper_library_flow_control/shifter_unit  data_width=1  pin_offset=5
      settings: SourceProductName=CASPER DSP Blockset
  shifter_unit7 : casper_library_flow_control/shifter_unit  data_width=1  pin_offset=6
      settings: SourceProductName=CASPER DSP Blockset
  shifter_unit8 : casper_library_flow_control/shifter_unit  data_width=1  pin_offset=7
      settings: SourceProductName=CASPER DSP Blockset
  shifter_unit9 : casper_library_flow_control/shifter_unit  data_width=1  pin_offset=8
      settings: SourceProductName=CASPER DSP Blockset
  sout : Outport
  wires:
  shifter_unit17/1 -> sout/1
  shifter_unit16/1 -> shifter_unit17/2
  shifter_unit15/1 -> shifter_unit16/2
  shifter_unit14/1 -> shifter_unit15/2
  shifter_unit13/1 -> shifter_unit14/2
  shifter_unit12/1 -> shifter_unit13/2
  shifter_unit11/1 -> shifter_unit12/2
  shifter_unit10/1 -> shifter_unit11/2
  shifter_unit9/1 -> shifter_unit10/2
  shifter_unit8/1 -> shifter_unit9/2
  shifter_unit7/1 -> shifter_unit8/2
  shifter_unit6/1 -> shifter_unit7/2
  shifter_unit5/1 -> shifter_unit6/2
  shifter_unit4/1 -> shifter_unit5/2
  shifter_unit3/1 -> shifter_unit4/2
  shifter_unit2/1 -> shifter_unit3/2
  shifter_unit1/1 -> shifter_unit2/2
  Logical/1 -> shifter_unit17/4, shifter_unit16/4, shifter_unit15/4, shifter_unit14/4, shifter_unit13/4, shifter_unit12/4, shifter_unit11/4, shifter_unit10/4, shifter_unit9/4, shifter_unit8/4, shifter_unit7/4, shifter_unit6/4, shifter_unit5/4, shifter_unit4/4, shifter_unit3/4, shifter_unit2/4, shifter_unit1/4
  pin/1 -> shifter_unit17/3, shifter_unit16/3, shifter_unit15/3, shifter_unit14/3, shifter_unit13/3, shifter_unit12/3, shifter_unit11/3, shifter_unit10/3, shifter_unit9/3, shifter_unit8/3, shifter_unit7/3, shifter_unit6/3, shifter_unit5/3, shifter_unit4/3, shifter_unit3/3, shifter_unit2/3, shifter_unit1/3
  filler/1 -> shifter_unit1/2
  shift/1 -> Logical/2
  ld/1 -> shifter_unit17/1, shifter_unit16/1, shifter_unit15/1, shifter_unit14/1, shifter_unit13/1, shifter_unit12/1, shifter_unit11/1, shifter_unit10/1, shifter_unit9/1, shifter_unit8/1, shifter_unit7/1, shifter_unit6/1, shifter_unit5/1, shifter_unit4/1, shifter_unit3/1, shifter_unit2/1, shifter_unit1/1, Logical/1
